simulink model "write"  (R2020a)
settings: Solver=VariableStepAuto  StartTime=0.0  StopTime=10.0  RelTol=1e-3
model workspace (MAT data in the model file):
  a = arduino
settings Model: OrderedModelArguments=off  Creator=mahmo  LastModifiedBy=mahmo

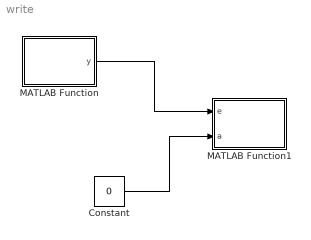
== system write ==
  Constant : Constant  Value=0
  MATLAB Function : MATLAB Function  TreatAsAtomicUnit=on
  MATLAB Function1 : MATLAB Function  TreatAsAtomicUnit=on
  wires:
  MATLAB Function/1(y) -> MATLAB Function1/1(e)
  Constant/1 -> MATLAB Function1/2(a)

== matlab function write/MATLAB Function ==
  data: y output
function y =fcn()


y=arduino('COM6');

== matlab function write/MATLAB Function1 ==
  data: e input; a input
function y(e,a)

writeDigitalPin(e,'D13',a);
